simulink model "spm"  (Simulink 7.6)
settings: Solver=ode4  StartTime=0.0  StopTime=.05  FixedStep=1e-6  RelTol=1e-4
undefined symbols (not defined in the file): pp
libraries: powerlib x15, simulink x4
settings Model: Creator=PhuongLe  LastModifiedBy=PhuongLe
settings SolverCC: SolverResetMethod=Robust

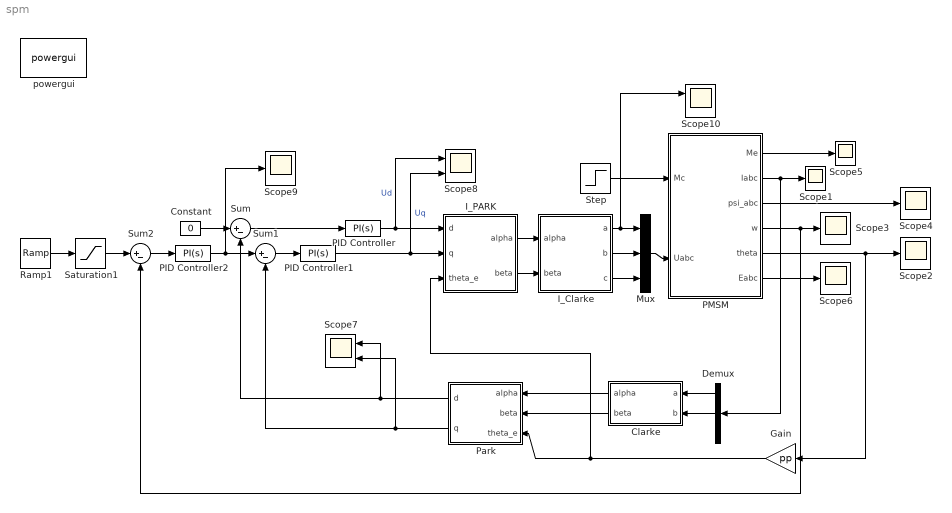
== system spm ==
  Clarke : Stateflow chart  TreatAsAtomicUnit=on
  Constant : Constant  Value=0
  Demux : Demux  Outputs=3
  Gain : Gain  Gain=pp
  I_Clarke : Stateflow chart  TreatAsAtomicUnit=on
  I_PARK : Stateflow chart  TreatAsAtomicUnit=on
  Mux : Mux  Inputs=3
  PID Controller : simulink/Continuous/PID Controller  DialogController=pidpack.PIDConfig.pidDDGCreate  DialogControllerArgs=DataTag0  SystemSampleTime=-1  Controller=PI  TimeDomain=Continuous-time  SampleTime=1  IntegratorMethod=Forward Euler  FilterMethod=Forward Euler  Form=Parallel  P=1000  I=.2  D=0  N=100  InitialConditionSource=internal  InitialConditionForIntegrator=0  InitialConditionForFilter=0  ExternalReset=none  LimitOutput=on  UpperSaturationLimit=80  LowerSaturationLimit=-80  LinearizeAsGain=off  AntiWindupMode=none  Kb=1  TrackingMode=off  Kt=1  PParamMin=[]  PParamMax=[]  IParamMin=[]  IParamMax=[]  DParamMin=[]  DParamMax=[]  NParamMin=[]  NParamMax=[]  KbParamMin=[]  KbParamMax=[]  KtParamMin=[]  KtParamMax=[]  POutMin=[]  POutMax=[]  IOutMin=[]  IOutMax=[]  DOutMin=[]  DOutMax=[]  NOutMin=[]  NOutMax=[]  KbOutMin=[]  KbOutMax=[]  KtOutMin=[]  KtOutMax=[]  IntegratorOutMin=[]  IntegratorOutMax=[]  FilterOutMin=[]  FilterOutMax=[]  SumOutMin=[]  SumOutMax=[]  SumI1OutMin=[]  SumI1OutMax=[]  SumI2OutMin=[]  SumI2OutMax=[]  SumI3OutMin=[]  SumI3OutMax=[]  SumDOutMin=[]  SumDOutMax=[]  SaturationOutMin=[]  SaturationOutMax=[]  IntegratorContinuousStateAttributes=''  IntegratorStateMustResolveToSignalObject=off  IntegratorRTWStateStorageClass=Auto  FilterContinuousStateAttributes=''  FilterStateMustResolveToSignalObject=off  FilterRTWStateStorageClass=Auto
  PID Controller1 : simulink/Continuous/PID Controller  DialogController=pidpack.PIDConfig.pidDDGCreate  DialogControllerArgs=DataTag1  SystemSampleTime=-1  Controller=PI  TimeDomain=Continuous-time  SampleTime=1  IntegratorMethod=Forward Euler  FilterMethod=Forward Euler  Form=Parallel  P=1000  I=.2  D=0  N=100  InitialConditionSource=internal  InitialConditionForIntegrator=0  InitialConditionForFilter=0  ExternalReset=none  LimitOutput=on  UpperSaturationLimit=200  LowerSaturationLimit=-200  LinearizeAsGain=off  AntiWindupMode=none  Kb=1  TrackingMode=off  Kt=1  PParamMin=[]  PParamMax=[]  IParamMin=[]  IParamMax=[]  DParamMin=[]  DParamMax=[]  NParamMin=[]  NParamMax=[]  KbParamMin=[]  KbParamMax=[]  KtParamMin=[]  KtParamMax=[]  POutMin=[]  POutMax=[]  IOutMin=[]  IOutMax=[]  DOutMin=[]  DOutMax=[]  NOutMin=[]  NOutMax=[]  KbOutMin=[]  KbOutMax=[]  KtOutMin=[]  KtOutMax=[]  IntegratorOutMin=[]  IntegratorOutMax=[]  FilterOutMin=[]  FilterOutMax=[]  SumOutMin=[]  SumOutMax=[]  SumI1OutMin=[]  SumI1OutMax=[]  SumI2OutMin=[]  SumI2OutMax=[]  SumI3OutMin=[]  SumI3OutMax=[]  SumDOutMin=[]  SumDOutMax=[]  SaturationOutMin=[]  SaturationOutMax=[]  IntegratorContinuousStateAttributes=''  IntegratorStateMustResolveToSignalObject=off  IntegratorRTWStateStorageClass=Auto  FilterContinuousStateAttributes=''  FilterStateMustResolveToSignalObject=off  FilterRTWStateStorageClass=Auto
  PID Controller2 : simulink/Continuous/PID Controller  DialogController=pidpack.PIDConfig.pidDDGCreate  DialogControllerArgs=DataTag2  SystemSampleTime=-1  Controller=PI  TimeDomain=Continuous-time  SampleTime=1  IntegratorMethod=Forward Euler  FilterMethod=Forward Euler  Form=Parallel  P=20  I=.005  D=0  N=100  InitialConditionSource=internal  InitialConditionForIntegrator=0  InitialConditionForFilter=0  ExternalReset=none  LimitOutput=on  UpperSaturationLimit=400  LowerSaturationLimit=-400  LinearizeAsGain=off  AntiWindupMode=none  Kb=1  TrackingMode=off  Kt=1  PParamMin=[]  PParamMax=[]  IParamMin=[]  IParamMax=[]  DParamMin=[]  DParamMax=[]  NParamMin=[]  NParamMax=[]  KbParamMin=[]  KbParamMax=[]  KtParamMin=[]  KtParamMax=[]  POutMin=[]  POutMax=[]  IOutMin=[]  IOutMax=[]  DOutMin=[]  DOutMax=[]  NOutMin=[]  NOutMax=[]  KbOutMin=[]  KbOutMax=[]  KtOutMin=[]  KtOutMax=[]  IntegratorOutMin=[]  IntegratorOutMax=[]  FilterOutMin=[]  FilterOutMax=[]  SumOutMin=[]  SumOutMax=[]  SumI1OutMin=[]  SumI1OutMax=[]  SumI2OutMin=[]  SumI2OutMax=[]  SumI3OutMin=[]  SumI3OutMax=[]  SumDOutMin=[]  SumDOutMax=[]  SaturationOutMin=[]  SaturationOutMax=[]  IntegratorContinuousStateAttributes=''  IntegratorStateMustResolveToSignalObject=off  IntegratorRTWStateStorageClass=Auto  FilterContinuousStateAttributes=''  FilterStateMustResolveToSignalObject=off  FilterRTWStateStorageClass=Auto
  PMSM : Subsystem  mask{R=0.228670895246976, pp=3, closestate=1, id_values=[-113.137084989848 -101.823376490863 -90.5096679918782 -79.1959594928934 -67.8822509939085 -56.5685424949238 -45.254833995939 -33.9411254969543 -22.6274169979695 -11.3137084989848 0 11.3137084989848 22.6274169979695 33.9411254969543 45.254833995939 56.5685424949238 67.8822509939085 79.1959594928934 90.5096679918782 101.823376490863 113.137084989848 ], psid_values=[0.172740632102786 0.18733841173438 0.202002774263266 0.216690300422651 0.231358784471999 0.245964711828234 0.260383456313227 0.274372331078355 0.287814279610171 0.300724209882799 0.31311684760952 0.324975495395059 0.336020337344254 0.345921274387856 0.354671703304871 0.362337854980303 0.368929918774175 0.374658567192816 0.379793052896991 0.38449824897862 0.388872468295376 ], iq_values=[-113.137084989848 -101.823376490863 -90.5096679918782 -79.1959594928935 -67.8822509939085 -56.5685424949238 -45.254833995939 -33.9411254969543 -22.6274169979695 -11.3137084989848 0 11.3137084989848 22.6274169979695 33.9411254969543 45.254833995939 56.5685424949238 67.8822509939085 79.1959594928935 90.5096679918782 101.823376490863 113.137084989848 ], psiq_values=[-0.112740389147521 -0.103477361864373 -0.0939890683250747 -0.084231724320993 -0.0740952334758474 -0.0633602527739227 -0.0518878214777416 -0.0397846483294785 -0.0270503725956554 -0.0136961509232942 -5.10904676949882E-06 0.0138121183329056 0.0277897687210442 0.0418840827815811 0.0560401844161457 0.0702357680771829 0.0844422061839439 0.098633550522013 0.112796914218953 0.126905250098708 0.140924953095323 ], J=5e-3, Fr=1e-5, w0=0, theta0=0}
      mask prompts: R "Resistance of phase"; pp "Pairs of poles"; closestate "Connect to power? (0-no,1-yes)"; id_values "Current d values"; psid_values "Fluxlinkage d values"; iq_values "Current q values"; psiq_values "Fluxlinkage q values"; J "Inertia"; Fr "Air resistance"; w0 "Initial speed (rad/s)"; theta0 "Initial position (rad)"
      mask TabNameString: Electrical,Electrical,Electrical,Electrical,Electrical,Electrical,Electrical,Mechanical,Mechanical,Mechanical,Mechanical
  Park : Stateflow chart  TreatAsAtomicUnit=on
  Ramp1 : simulink/Sources/Ramp  SystemSampleTime=-1  slope=5000  start=0  X0=0
  Saturation1 : Saturate  UpperLimit=100  LowerLimit=0
  Scope{1..6,9} (7 alike) : Scope
      Scope2 settings: SaveName=ScopeData3
      Scope3 settings: TimeRange=0.2  YMin=92.9725  YMax=102.759  SaveName=ScopeData6
      Scope4 settings: TimeRange=0.01  SaveName=ScopeData7
      Scope5 settings: YMin=0  YMax=90  SaveName=ScopeData8
      Scope6 settings: SaveName=ScopeData9
      Scope9 settings: TimeRange=0.2  YMin=0  YMax=80  SaveName=ScopeData14
  Scope10 : Scope  NumInputPorts=2
      settings: TimeRange=0.2  YMin=-250~-1  YMax=250~1  SaveName=ScopeData15
  Scope7 : Scope  NumInputPorts=2
      settings: TimeRange=0.2  YMin=-0.0025~0  YMax=0.02~60  SaveName=ScopeData10
  Scope8 : Scope  NumInputPorts=2
      settings: TimeRange=0.2  YMin=-5~-5  YMax=5~5  SaveName=ScopeData13
  Step : Step  Time=.03  After=80  SampleTime=0
  Sum : Sum  Inputs=|+-
  Sum1 : Sum  Inputs=|+-
  Sum2 : Sum  Inputs=|+-
  powergui : powerlib/powergui  Priority=1  SystemSampleTime=-1  SimulationMode=Continuous  SampleTime=50e-6  frequency=60  SPID=off  DisableSnubberDevices=off  DisableRonSwitches=off  DisableVfSwitches=off  SwTol=0  Interpol=off  frequencyindice=0  echomessages=off  HookPort=off  DisplayEquations=off  FunctionMessages=off  EnableUseOfTLC=off  x0status=blocks  RestoreLinks=warning  ResistiveCurrentMeasurement=off  Ylog=off  Xlog=on  ShowGrid=off  save=off  variable=ZData  ZoomFFT=off  StartTime=0.0  cycles=1  DisplayStyle=1  FreqAxis=off  MaxFrequency=1000  frequencyindicesteady=1  display=off  methode=off
  wires:
  PMSM/2(Iabc) -> Scope1/1, Demux/1
  PMSM/5(theta) -> Scope2/1, Gain/1
  PMSM/4(w) -> Scope3/1, Sum2/2
  PMSM/3(psi_abc) -> Scope4/1
  PMSM/1(Me) -> Scope5/1
  PMSM/6(Eabc) -> Scope6/1
  Step/1 -> PMSM/1(Mc)
  Clarke/1(alpha) -> Park/1(alpha)
  Clarke/2(beta) -> Park/2(beta)
  Demux/1 -> Clarke/1(a)
  Demux/2 -> Clarke/2(b)
  Gain/1 -> Park/3(theta_e), I_PARK/3(theta_e)
  Mux/1 -> PMSM/2(Uabc)
  I_Clarke/1(a) -> Mux/1, Scope10/1
  I_Clarke/2(b) -> Mux/2
  I_Clarke/3(c) -> Mux/3
  I_PARK/1(alpha) -> I_Clarke/1(alpha)
  I_PARK/2(beta) -> I_Clarke/2(beta)
  Park/1(d) -> Sum/2, Scope7/1
  Park/2(q) -> Sum1/2, Scope7/2
  Constant/1 -> Sum/1
  Sum1/1 -> PID Controller1/1
  PID Controller1/1 -> I_PARK/2(q), Scope8/2  "Uq"
  Sum/1 -> PID Controller/1
  PID Controller/1 -> I_PARK/1(d), Scope8/1  "Ud"
  Sum2/1 -> PID Controller2/1
  Ramp1/1 -> Saturation1/1
  Saturation1/1 -> Sum2/1
  PID Controller2/1 -> Sum1/1, Scope9/1

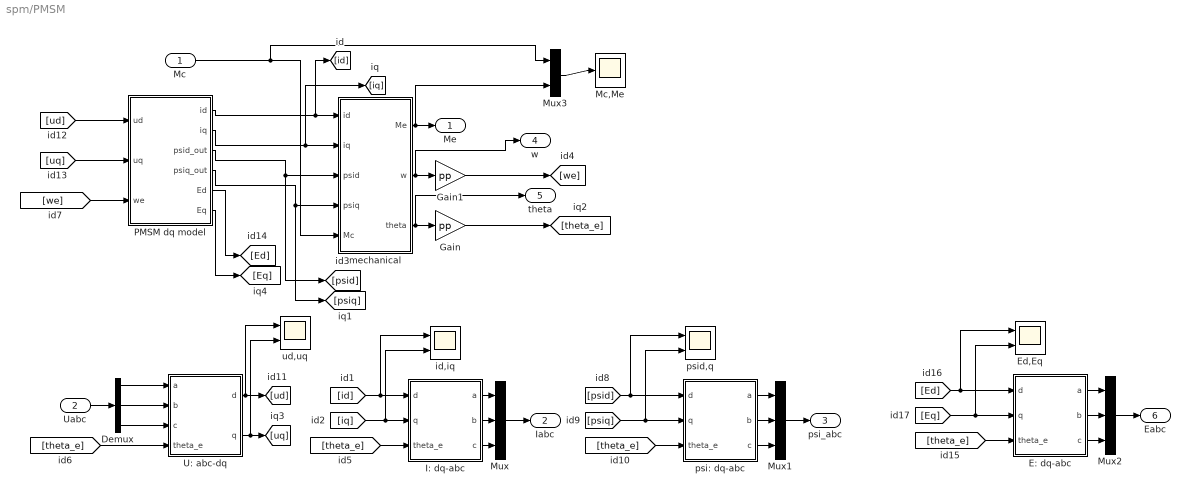
== system spm/PMSM ==
  Mc : Inport
  Uabc : Inport  Port=2
  Demux : Demux  Outputs=3
  E: dq-abc : Subsystem
  Ed,Eq : Scope  NumInputPorts=2
      settings: YMin=-5~-5  YMax=5~5
  Gain : Gain  Gain=pp
  Gain1 : Gain  Gain=pp
  I: dq-abc : Subsystem
  Mc,Me : Scope
      settings: SaveName=ScopeData12
  Mux : Mux  Inputs=3
  Mux1 : Mux  Inputs=3
  Mux2 : Mux  Inputs=3
  Mux3 : Mux  Inputs=2
  PMSM dq model : Subsystem
  U: abc-dq : Subsystem
  id,iq : Scope  NumInputPorts=2
      settings: YMin=-5~-5  YMax=5~5  SaveName=ScopeData4
  mechanical : Subsystem
  psi: dq-abc : Subsystem
  psid,q : Scope  NumInputPorts=2
      settings: YMin=-5~-5  YMax=5~5  SaveName=ScopeData5
  ud,uq : Scope  NumInputPorts=2
      settings: YMin=-5~-5  YMax=5~5  SaveName=ScopeData2
  Me : Outport
  Iabc : Outport  Port=2
  psi_abc : Outport  Port=3
  w : Outport  Port=4
  theta : Outport  Port=5
  Eabc : Outport  Port=6
  wires:
  [uq] -> PMSM dq model/2(uq)
  [ud] -> PMSM dq model/1(ud)
  mechanical/3(theta) -> Gain/1, theta/1
  Gain/1 -> [theta_e]
  mechanical/2(w) -> Gain1/1, w/1
  Gain1/1 -> [we]
  PMSM dq model/1(id) -> mechanical/1(id), [id]
  PMSM dq model/2(iq) -> mechanical/2(iq), [iq]
  PMSM dq model/3(psid_out) -> mechanical/3(psid), [psid]
  PMSM dq model/4(psiq_out) -> mechanical/4(psiq), [psiq]
  [id] -> I: dq-abc/1(d), id,iq/1
  [iq] -> I: dq-abc/2(q), id,iq/2
  [theta_e] -> I: dq-abc/3(theta_e)
  [we] -> PMSM dq model/3(we)
  [psid] -> psi: dq-abc/1(d), psid,q/1
  [psiq] -> psi: dq-abc/2(q), psid,q/2
  [theta_e] -> psi: dq-abc/3(theta_e)
  [theta_e] -> U: abc-dq/4(theta_e)
  U: abc-dq/1(d) -> [ud], ud,uq/1
  U: abc-dq/2(q) -> [uq], ud,uq/2
  I: dq-abc/1(a) -> Mux/1
  I: dq-abc/2(b) -> Mux/2
  I: dq-abc/3(c) -> Mux/3
  psi: dq-abc/1(a) -> Mux1/1
  psi: dq-abc/2(b) -> Mux1/2
  psi: dq-abc/3(c) -> Mux1/3
  Demux/1 -> U: abc-dq/1(a)
  Demux/2 -> U: abc-dq/2(b)
  Demux/3 -> U: abc-dq/3(c)
  mechanical/1(Me) -> Me/1, Mux3/2
  Mc/1 -> mechanical/5(Mc), Mux3/1
  Uabc/1 -> Demux/1
  Mux/1 -> Iabc/1
  Mux1/1 -> psi_abc/1
  PMSM dq model/5(Ed) -> [Ed]
  PMSM dq model/6(Eq) -> [Eq]
  [Ed] -> Ed,Eq/1, E: dq-abc/1(d)
  [Eq] -> Ed,Eq/2, E: dq-abc/2(q)
  [theta_e] -> E: dq-abc/3(theta_e)
  E: dq-abc/1(a) -> Mux2/1
  E: dq-abc/2(b) -> Mux2/2
  E: dq-abc/3(c) -> Mux2/3
  Mux2/1 -> Eabc/1
  Mux3/1 -> Mc,Me/1

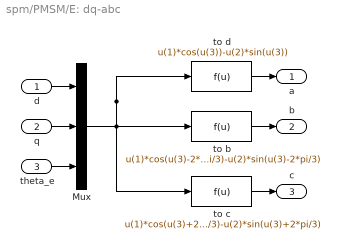
== system spm/PMSM/E: dq-abc ==
  d : Inport
  q : Inport  Port=2
  theta_e : Inport  Port=3
  Mux : Mux  Inputs=3
  to b : Fcn  Expr=u(1)*cos(u(3)-2*pi/3)-u(2)*sin(u(3)-2*pi/3)
  to c : Fcn  Expr=u(1)*cos(u(3)+2*pi/3)-u(2)*sin(u(3)+2*pi/3)
  to d : Fcn  Expr=u(1)*cos(u(3))-u(2)*sin(u(3))
  a : Outport
  b : Outport  Port=2
  c : Outport  Port=3
  wires:
  to c/1 -> c/1
  theta_e/1 -> Mux/3
  to b/1 -> b/1
  q/1 -> Mux/2
  to d/1 -> a/1
  d/1 -> Mux/1
  Mux/1 -> to c/1, to b/1, to d/1

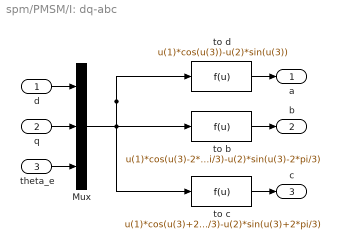
== system spm/PMSM/I: dq-abc ==
  d : Inport
  q : Inport  Port=2
  theta_e : Inport  Port=3
  Mux : Mux  Inputs=3
  to b : Fcn  Expr=u(1)*cos(u(3)-2*pi/3)-u(2)*sin(u(3)-2*pi/3)
  to c : Fcn  Expr=u(1)*cos(u(3)+2*pi/3)-u(2)*sin(u(3)+2*pi/3)
  to d : Fcn  Expr=u(1)*cos(u(3))-u(2)*sin(u(3))
  a : Outport
  b : Outport  Port=2
  c : Outport  Port=3
  wires:
  Mux/1 -> to d/1, to b/1, to c/1
  d/1 -> Mux/1
  to d/1 -> a/1
  q/1 -> Mux/2
  to b/1 -> b/1
  theta_e/1 -> Mux/3
  to c/1 -> c/1

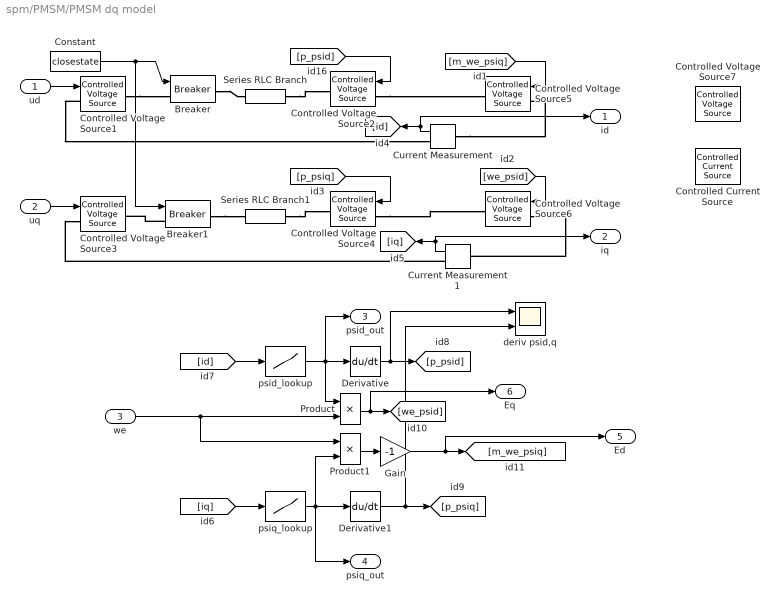
== system spm/PMSM/PMSM dq model ==
  ud : Inport
  uq : Inport  Port=2
  we : Inport  Port=3
  Breaker : powerlib/Elements/Breaker  DialogController=POWERSYS.PowerSysDialog  SystemSampleTime=-1  BreakerResistance=1e-3  InitialState=closestate  SnubberResistance=1e9  SnubberCapacitance=inf  SwitchingTimes="[ 1/60  5/60 ]"  External=on  Measurements=None  MoreParameters=off  NoBreakLoop=off
  Breaker1 : powerlib/Elements/Breaker  DialogController=POWERSYS.PowerSysDialog  SystemSampleTime=-1  BreakerResistance=1e-3  InitialState=closestate  SnubberResistance=1e9  SnubberCapacitance=inf  SwitchingTimes="[ 1/60  5/60 ]"  External=on  Measurements=None  MoreParameters=off  NoBreakLoop=off
  Constant : Constant  Value=closestate
  Controlled Current Source : powerlib/Electrical Sources/Controlled Current Source  DialogController=POWERSYS.PowerSysDialog  SystemSampleTime=-1  Initialize=on  Source_Type=AC  Amplitude=0  Phase=0  Frequency=0  Measurements=None
  Controlled Voltage Source{1..7} (7 alike) : powerlib/Electrical Sources/Controlled Voltage Source  DialogController=POWERSYS.PowerSysDialog  SystemSampleTime=-1  Initialize=off  Source_Type=DC  Amplitude=0  Phase=0  Frequency=0  Measurements=None
  Current Measurement : powerlib/Measurements/Current Measurement  DialogController=POWERSYS.PowerSysDialog  SystemSampleTime=-1  PhasorSimulation=off  OutputType=Complex  PSBequivalent=0
      link override source: GotoTag=tpb8be4e0b_b0e5_4bc5_b433_21e872ee0d69
  Current Measurement1 : powerlib/Measurements/Current Measurement  DialogController=POWERSYS.PowerSysDialog  SystemSampleTime=-1  PhasorSimulation=off  OutputType=Complex  PSBequivalent=0
  Derivative : Derivative
  Derivative1 : Derivative
  Gain : Gain  Gain=-1
  Product : Product  RndMeth=Zero
  Product1 : Product  RndMeth=Zero
  Series RLC Branch : powerlib/Elements/Series RLC Branch  DialogController=POWERSYS.PowerSysDialog  PhysicalDomain=powersysdomain  SubClassName=unknown  LeftPortType=p1  RightPortType=p1  LConnTagsString=__new0  RConnTagsString=__new0  BranchType=R  Resistance=R  Inductance=1e-3  SetiL0=off  InitialCurrent=0  Capacitance=1e-6  Setx0=off  InitialVoltage=0  Measurements=None
  Series RLC Branch1 : powerlib/Elements/Series RLC Branch  DialogController=POWERSYS.PowerSysDialog  PhysicalDomain=powersysdomain  SubClassName=unknown  LeftPortType=p1  RightPortType=p1  LConnTagsString=__new0  RConnTagsString=__new0  BranchType=R  Resistance=R  Inductance=1e-3  SetiL0=off  InitialCurrent=0  Capacitance=1e-6  Setx0=off  InitialVoltage=0  Measurements=None
  deriv psid,q : Scope  NumInputPorts=2
      settings: YMin=-5~-5  YMax=5~5  SaveName=ScopeData11
  psid_lookup : Lookup  InputValues=id_values  Table=psid_values
  psiq_lookup : Lookup  InputValues=iq_values  Table=psiq_values
  id : Outport
  iq : Outport  Port=2
  psid_out : Outport  Port=3
  psiq_out : Outport  Port=4
  Ed : Outport  Port=5
  Eq : Outport  Port=6
  wires:
  psiq_lookup/1 -> Derivative1/1, Product1/2, psiq_out/1
  [p_psid] -> Controlled Voltage Source2/1
  [m_we_psiq] -> Controlled Voltage Source5/1
  ud/1 -> Controlled Voltage Source1/1
  [p_psiq] -> Controlled Voltage Source4/1
  [we_psid] -> Controlled Voltage Source6/1
  uq/1 -> Controlled Voltage Source3/1
  Current Measurement/1 -> [id], id/1
  Current Measurement1/1 -> [iq], iq/1
  [iq] -> psiq_lookup/1
  psid_lookup/1 -> Derivative/1, Product/1, psid_out/1
  [id] -> psid_lookup/1
  Derivative/1 -> [p_psid], deriv psid,q/1
  Derivative1/1 -> [p_psiq], deriv psid,q/2
  we/1 -> Product/2, Product1/1
  Product/1 -> [we_psid], Eq/1
  Product1/1 -> Gain/1
  Constant/1 -> Breaker/1, Breaker1/1
  Gain/1 -> [m_we_psiq], Ed/1
  connections:
  Series RLC Branch/RConn1 -- Controlled Voltage Source2/RConn1
  Controlled Voltage Source2/LConn1 -- Controlled Voltage Source5/RConn1
  Current Measurement1/RConn1 -- Controlled Voltage Source3/LConn1
  Series RLC Branch1/RConn1 -- Controlled Voltage Source4/RConn1
  Controlled Voltage Source4/LConn1 -- Controlled Voltage Source6/RConn1
  Current Measurement/LConn1 -- Controlled Voltage Source5/LConn1
  Controlled Voltage Source6/LConn1 -- Current Measurement1/LConn1
  Controlled Voltage Source1/LConn1 -- Current Measurement/RConn1
  Breaker/RConn1 -- Series RLC Branch/LConn1
  Controlled Voltage Source1/RConn1 -- Breaker/LConn1
  Breaker1/RConn1 -- Series RLC Branch1/LConn1
  Breaker1/LConn1 -- Controlled Voltage Source3/RConn1

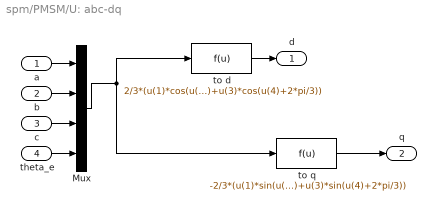
== system spm/PMSM/U: abc-dq ==
  a : Inport
  b : Inport  Port=2
  c : Inport  Port=3
  theta_e : Inport  Port=4
  Mux : Mux
  to d : Fcn  Expr=2/3*(u(1)*cos(u(4))+u(2)*cos(u(4)-2*pi/3)+u(3)*cos(u(4)+2*pi/3))
  to q : Fcn  Expr=-2/3*(u(1)*sin(u(4))+u(2)*sin(u(4)-2*pi/3)+u(3)*sin(u(4)+2*pi/3))
  d : Outport
  q : Outport  Port=2
  wires:
  Mux/1 -> to d/1, to q/1
  a/1 -> Mux/1
  to d/1 -> d/1
  b/1 -> Mux/2
  c/1 -> Mux/3
  to q/1 -> q/1
  theta_e/1 -> Mux/4

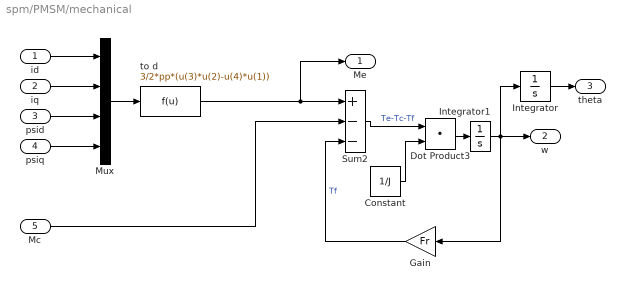
== system spm/PMSM/mechanical ==
  id : Inport
  iq : Inport  Port=2
  psid : Inport  Port=3
  psiq : Inport  Port=4
  Mc : Inport  Port=5
  Constant : Constant  Value=1/J
  Dot Product3 : DotProduct  InputSameDT=on  OutDataTypeStr=Inherit: Inherit via internal rule
  Gain : Gain  Gain=Fr
  Integrator : Integrator  InitialCondition=theta0
  Integrator1 : Integrator  InitialCondition=w0
  Mux : Mux
  Sum2 : Sum  Inputs=+--
  to d : Fcn  Expr=3/2*pp*(u(3)*u(2)-u(4)*u(1))
  Me : Outport
  w : Outport  Port=2
  theta : Outport  Port=3
  wires:
  Mc/1 -> Sum2/2
  Sum2/1 -> Dot Product3/1  "Te-Tc-Tf"
  Constant/1 -> Dot Product3/2
  Dot Product3/1 -> Integrator1/1
  Gain/1 -> Sum2/3  "Tf"
  Integrator/1 -> theta/1
  Integrator1/1 -> w/1, Gain/1, Integrator/1
  to d/1 -> Sum2/1, Me/1
  id/1 -> Mux/1
  iq/1 -> Mux/2
  psid/1 -> Mux/3
  psiq/1 -> Mux/4
  Mux/1 -> to d/1

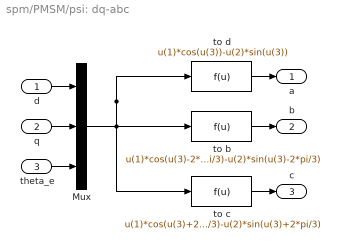
== system spm/PMSM/psi: dq-abc ==
  d : Inport
  q : Inport  Port=2
  theta_e : Inport  Port=3
  Mux : Mux  Inputs=3
  to b : Fcn  Expr=u(1)*cos(u(3)-2*pi/3)-u(2)*sin(u(3)-2*pi/3)
  to c : Fcn  Expr=u(1)*cos(u(3)+2*pi/3)-u(2)*sin(u(3)+2*pi/3)
  to d : Fcn  Expr=u(1)*cos(u(3))-u(2)*sin(u(3))
  a : Outport
  b : Outport  Port=2
  c : Outport  Port=3
  wires:
  Mux/1 -> to d/1, to b/1, to c/1
  d/1 -> Mux/1
  to d/1 -> a/1
  q/1 -> Mux/2
  to b/1 -> b/1
  theta_e/1 -> Mux/3
  to c/1 -> c/1

== matlab function Park ==
  data: alpha input double; beta input double; theta_e input double; d output double; q output double
function [d,q] = fcn(alpha,beta,theta_e)
%#eml
d = alpha*cos(theta_e)+beta*sin(theta_e);
q = -alpha*sin(theta_e)+beta*cos(theta_e);

== matlab function Clarke ==
  data: a input double; alpha output double; b input double; beta output double
function [alpha,beta] = fcn(a,b)
%#eml
alpha = a;
beta = (2*b+a)/sqrt(3);

== matlab function I_PARK ==
  data: d input double; q input double; alpha output double; beta output double; theta_e input double
function [alpha,beta] = fcn(d,q,theta_e)
%#eml
alpha = d*cos(theta_e)-q*sin(theta_e);
beta = d*sin(theta_e)+q*cos(theta_e);

== matlab function I_Clarke ==
  data: alpha input double; beta input double; a output double; b output double; c output double
function [a,b,c] = fcn(alpha,beta)
%#eml
a = alpha;
b = -alpha/2+sqrt(3)/2*beta;
c = -alpha/2-sqrt(3)/2*beta;
